simulink model "prj_2018a"  (R2018a)
settings: Solver=FixedStepAuto  StartTime=0.0  StopTime=T  FixedStep=0.01  RelTol=1e-3
values from neighbouring files (symbols this model uses):
  C0 = 0.008    [data.m]
  C1 = 1.6e-6    (= 1.6e-06)    [data.m]
  Cbat = 800    [data.m]
  Cx = 1.2    [data.m]
  D = 3    [data.m]
  g = 9.81    [data.m]
  m = 3    [data.m]
  rho = 1.225    [data.m]
  S = 0.0739    [data.m]
  T = 600    [data.m]
  VBAT = 12    [data.m]
libraries: simulink x3, powerlib_meascontrol x1
settings Model: Creator=xoxox  LastModifiedBy=eduhamel01
settings DataIOCC: ReturnWorkspaceOutputs=on
settings SFSimCC: SimUseLocalCustomCode=on
settings RTWCC: RTWUseLocalCustomCode=on

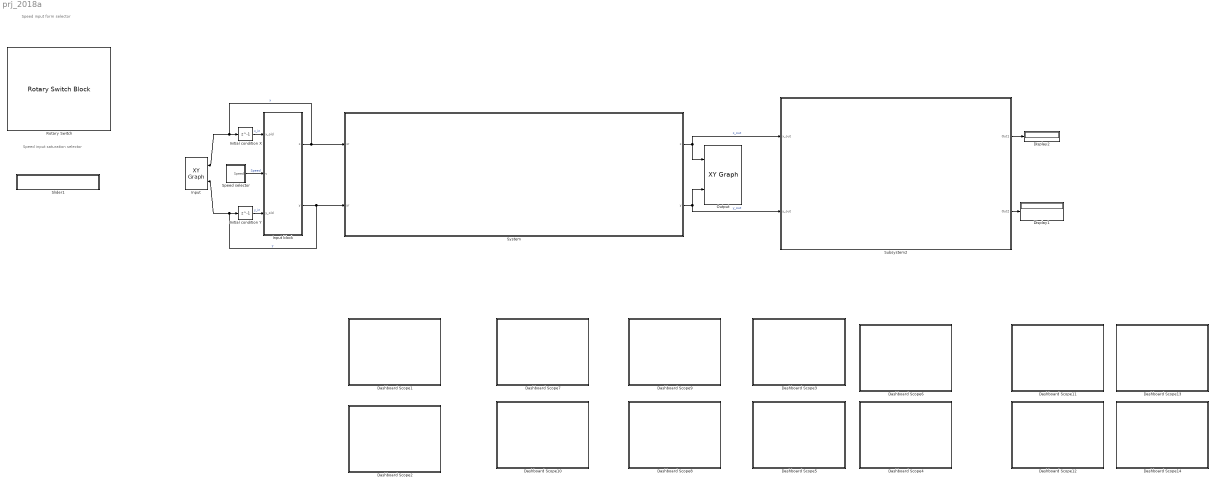
== system prj_2018a ==
  note: Speed input saturation
      | selector
  note: Speed input form selector
  Dashboard Scope1 : Subsystem  DialogController=hmiCreateDDGDialog  IsWebBlock=on  mask(MWDashboardBlock){webBlockId=119e8fbf-0f84-4c64-a065-49c5137ac74d, webBlockType=sdiscope, ShowInLibBrowser=on, ShowInitialText=on, HMISrcModelName=prj_2018a}
      mask prompts: webBlockId "WebBlock Id"; webBlockType "WebBlock Type"; HMISrcModelName "Source Model"
      mask help: Traces signals on the dashboard scope during simulation.
      mask Help: helpview([docroot '/mapfiles/simulink.map'], 'hmi_scope')
      mask Display:
      | if strcmp(get_param(bdroot(gcb),'BlockDiagramType'),'library')
      |  image([(matlabroot) '/toolbox/simulink/hmi/icons/SDIScope.png'])
      | end
  Dashboard Scope10 : Subsystem  DialogController=hmiCreateDDGDialog  IsWebBlock=on  mask(MWDashboardBlock){webBlockId=fa008d0d-197e-41b1-bb55-4dce241af62d, webBlockType=sdiscope, ShowInLibBrowser=on, ShowInitialText=on, HMISrcModelName=prj_2018a}
      mask prompts: webBlockId "WebBlock Id"; webBlockType "WebBlock Type"; HMISrcModelName "Source Model"
      mask help: Traces signals on the dashboard scope during simulation.
      mask Help: helpview([docroot '/mapfiles/simulink.map'], 'hmi_scope')
      mask Display:
      | if strcmp(get_param(bdroot(gcb),'BlockDiagramType'),'library')
      |  image([(matlabroot) '/toolbox/simulink/hmi/icons/SDIScope.png'])
      | end
  Dashboard Scope11 : Subsystem  DialogController=hmiCreateDDGDialog  IsWebBlock=on  mask(MWDashboardBlock){webBlockId=fa4fd851-4fca-4c18-b171-96f8acd06293, webBlockType=sdiscope, ShowInLibBrowser=on, ShowInitialText=on, HMISrcModelName=prj_2018a}
      mask prompts: webBlockId "WebBlock Id"; webBlockType "WebBlock Type"; HMISrcModelName "Source Model"
      mask help: Traces signals on the dashboard scope during simulation.
      mask Help: helpview([docroot '/mapfiles/simulink.map'], 'hmi_scope')
      mask Display:
      | if strcmp(get_param(bdroot(gcb),'BlockDiagramType'),'library')
      |  image([(matlabroot) '/toolbox/simulink/hmi/icons/SDIScope.png'])
      | end
  Dashboard Scope12 : Subsystem  DialogController=hmiCreateDDGDialog  IsWebBlock=on  mask(MWDashboardBlock){webBlockId=7913e7ce-348c-44da-9251-239d1fa42c28, webBlockType=sdiscope, ShowInLibBrowser=on, ShowInitialText=on, HMISrcModelName=prj_2018a}
      mask prompts: webBlockId "WebBlock Id"; webBlockType "WebBlock Type"; HMISrcModelName "Source Model"
      mask help: Traces signals on the dashboard scope during simulation.
      mask Help: helpview([docroot '/mapfiles/simulink.map'], 'hmi_scope')
      mask Display:
      | if strcmp(get_param(bdroot(gcb),'BlockDiagramType'),'library')
      |  image([(matlabroot) '/toolbox/simulink/hmi/icons/SDIScope.png'])
      | end
  Dashboard Scope13 : Subsystem  DialogController=hmiCreateDDGDialog  IsWebBlock=on  mask(MWDashboardBlock){webBlockId=8edd69cc-18a3-423d-a06d-795dad7adbdd, webBlockType=sdiscope, ShowInLibBrowser=on, ShowInitialText=on, HMISrcModelName=prj_2018a}
      mask prompts: webBlockId "WebBlock Id"; webBlockType "WebBlock Type"; HMISrcModelName "Source Model"
      mask help: Traces signals on the dashboard scope during simulation.
      mask Help: helpview([docroot '/mapfiles/simulink.map'], 'hmi_scope')
      mask Display:
      | if strcmp(get_param(bdroot(gcb),'BlockDiagramType'),'library')
      |  image([(matlabroot) '/toolbox/simulink/hmi/icons/SDIScope.png'])
      | end
  Dashboard Scope14 : Subsystem  DialogController=hmiCreateDDGDialog  IsWebBlock=on  mask(MWDashboardBlock){webBlockId=3235017e-418f-422e-8807-0662af4a4bf4, webBlockType=sdiscope, ShowInLibBrowser=on, ShowInitialText=on, HMISrcModelName=prj_2018a}
      mask prompts: webBlockId "WebBlock Id"; webBlockType "WebBlock Type"; HMISrcModelName "Source Model"
      mask help: Traces signals on the dashboard scope during simulation.
      mask Help: helpview([docroot '/mapfiles/simulink.map'], 'hmi_scope')
      mask Display:
      | if strcmp(get_param(bdroot(gcb),'BlockDiagramType'),'library')
      |  image([(matlabroot) '/toolbox/simulink/hmi/icons/SDIScope.png'])
      | end
  Dashboard Scope2 : Subsystem  DialogController=hmiCreateDDGDialog  IsWebBlock=on  mask(MWDashboardBlock){webBlockId=834b94e8-2ac5-4a88-9e83-ba3259317c2a, webBlockType=sdiscope, ShowInLibBrowser=on, ShowInitialText=on, HMISrcModelName=prj_2018a}
      mask prompts: webBlockId "WebBlock Id"; webBlockType "WebBlock Type"; HMISrcModelName "Source Model"
      mask help: Traces signals on the dashboard scope during simulation.
      mask Help: helpview([docroot '/mapfiles/simulink.map'], 'hmi_scope')
      mask Display:
      | if strcmp(get_param(bdroot(gcb),'BlockDiagramType'),'library')
      |  image([(matlabroot) '/toolbox/simulink/hmi/icons/SDIScope.png'])
      | end
  Dashboard Scope3 : Subsystem  DialogController=hmiCreateDDGDialog  IsWebBlock=on  mask(MWDashboardBlock){webBlockId=06c2f07c-ed11-4a51-95f8-aa5a8867ac83, webBlockType=sdiscope, ShowInLibBrowser=on, ShowInitialText=on, HMISrcModelName=prj_2018a}
      mask prompts: webBlockId "WebBlock Id"; webBlockType "WebBlock Type"; HMISrcModelName "Source Model"
      mask help: Traces signals on the dashboard scope during simulation.
      mask Help: helpview([docroot '/mapfiles/simulink.map'], 'hmi_scope')
      mask Display:
      | if strcmp(get_param(bdroot(gcb),'BlockDiagramType'),'library')
      |  image([(matlabroot) '/toolbox/simulink/hmi/icons/SDIScope.png'])
      | end
  Dashboard Scope4 : Subsystem  DialogController=hmiCreateDDGDialog  IsWebBlock=on  mask(MWDashboardBlock){webBlockId=6b045230-5b5a-4611-980b-31087ea3d308, webBlockType=sdiscope, ShowInLibBrowser=on, ShowInitialText=on, HMISrcModelName=prj_2018a}
      mask prompts: webBlockId "WebBlock Id"; webBlockType "WebBlock Type"; HMISrcModelName "Source Model"
      mask help: Traces signals on the dashboard scope during simulation.
      mask Help: helpview([docroot '/mapfiles/simulink.map'], 'hmi_scope')
      mask Display:
      | if strcmp(get_param(bdroot(gcb),'BlockDiagramType'),'library')
      |  image([(matlabroot) '/toolbox/simulink/hmi/icons/SDIScope.png'])
      | end
  Dashboard Scope5 : Subsystem  DialogController=hmiCreateDDGDialog  IsWebBlock=on  mask(MWDashboardBlock){webBlockId=d05e08e3-8fad-4b3c-942c-8af112444a54, webBlockType=sdiscope, ShowInLibBrowser=on, ShowInitialText=on, HMISrcModelName=prj_2018a}
      mask prompts: webBlockId "WebBlock Id"; webBlockType "WebBlock Type"; HMISrcModelName "Source Model"
      mask help: Traces signals on the dashboard scope during simulation.
      mask Help: helpview([docroot '/mapfiles/simulink.map'], 'hmi_scope')
      mask Display:
      | if strcmp(get_param(bdroot(gcb),'BlockDiagramType'),'library')
      |  image([(matlabroot) '/toolbox/simulink/hmi/icons/SDIScope.png'])
      | end
  Dashboard Scope6 : Subsystem  DialogController=hmiCreateDDGDialog  IsWebBlock=on  mask(MWDashboardBlock){webBlockId=a3c59839-8da6-40a2-abfa-24167c38daa9, webBlockType=sdiscope, ShowInLibBrowser=on, ShowInitialText=on, HMISrcModelName=prj_2018a}
      mask prompts: webBlockId "WebBlock Id"; webBlockType "WebBlock Type"; HMISrcModelName "Source Model"
      mask help: Traces signals on the dashboard scope during simulation.
      mask Help: helpview([docroot '/mapfiles/simulink.map'], 'hmi_scope')
      mask Display:
      | if strcmp(get_param(bdroot(gcb),'BlockDiagramType'),'library')
      |  image([(matlabroot) '/toolbox/simulink/hmi/icons/SDIScope.png'])
      | end
  Dashboard Scope7 : Subsystem  DialogController=hmiCreateDDGDialog  IsWebBlock=on  mask(MWDashboardBlock){webBlockId=a1a62eab-3a48-418c-ad90-13885701b78d, webBlockType=sdiscope, ShowInLibBrowser=on, ShowInitialText=on, HMISrcModelName=prj_2018a}
      mask prompts: webBlockId "WebBlock Id"; webBlockType "WebBlock Type"; HMISrcModelName "Source Model"
      mask help: Traces signals on the dashboard scope during simulation.
      mask Help: helpview([docroot '/mapfiles/simulink.map'], 'hmi_scope')
      mask Display:
      | if strcmp(get_param(bdroot(gcb),'BlockDiagramType'),'library')
      |  image([(matlabroot) '/toolbox/simulink/hmi/icons/SDIScope.png'])
      | end
  Dashboard Scope8 : Subsystem  DialogController=hmiCreateDDGDialog  IsWebBlock=on  mask(MWDashboardBlock){webBlockId=c0fb3f3b-45df-43b4-8987-c7cbfe6d8ce9, webBlockType=sdiscope, ShowInLibBrowser=on, ShowInitialText=on, HMISrcModelName=prj_2018a}
      mask prompts: webBlockId "WebBlock Id"; webBlockType "WebBlock Type"; HMISrcModelName "Source Model"
      mask help: Traces signals on the dashboard scope during simulation.
      mask Help: helpview([docroot '/mapfiles/simulink.map'], 'hmi_scope')
      mask Display:
      | if strcmp(get_param(bdroot(gcb),'BlockDiagramType'),'library')
      |  image([(matlabroot) '/toolbox/simulink/hmi/icons/SDIScope.png'])
      | end
  Dashboard Scope9 : Subsystem  DialogController=hmiCreateDDGDialog  IsWebBlock=on  mask(MWDashboardBlock){webBlockId=857b3752-856c-4ac0-8c31-3300ce0e1cd1, webBlockType=sdiscope, ShowInLibBrowser=on, ShowInitialText=on, HMISrcModelName=prj_2018a}
      mask prompts: webBlockId "WebBlock Id"; webBlockType "WebBlock Type"; HMISrcModelName "Source Model"
      mask help: Traces signals on the dashboard scope during simulation.
      mask Help: helpview([docroot '/mapfiles/simulink.map'], 'hmi_scope')
      mask Display:
      | if strcmp(get_param(bdroot(gcb),'BlockDiagramType'),'library')
      |  image([(matlabroot) '/toolbox/simulink/hmi/icons/SDIScope.png'])
      | end
  Display1 : Display
  Display2 : Display
  Initial condition X : Delay  DelayLength=1
  Initial condition Y : Delay  DelayLength=1
  Input : simulink/Sinks/XY Graph  xmin=-1  xmax=5.5  ymin=-5  ymax=20  st=-1
  Input block : MATLAB Function  TreatAsAtomicUnit=on
  Output : simulink/Sinks/XY Graph  xmin=-1  xmax=5.5  ymin=-5  ymax=20  st=-1
  Rotary Switch : RotarySwitchBlock  WebBlockId=65
      settings: Values={{'Constant', 'Sine', 'Pulse', 'Ramp', 'Triangle'}, [1 2 3 4 5]}
  Slider1 : Subsystem  DialogController=hmiCreateDDGDialog  IsWebBlock=on  mask(MWDashboardBlock){webBlockId=c1551613-8028-4e7c-bb00-03568ac3d875, webBlockType=slider, ShowInLibBrowser=on, ShowInitialText=on, HMISrcModelName=prj_2018a}
      mask prompts: webBlockId "WebBlock Id"; webBlockType "WebBlock Type"; HMISrcModelName "Source Model"
      mask help: Set value to tune parameters or variables.
      mask Help: helpview([docroot '/mapfiles/simulink.map'], 'hmi_slider')
      mask Display:
      | if strcmp(get_param(bdroot(gcb),'BlockDiagramType'),'library')
      |  image([(matlabroot) '/toolbox/simulink/hmi/icons/Slider.png'])
      | end
  Speed selector : Subsystem
  Subsystem2 : Subsystem
  System : Subsystem
  wires:
  System/1(x) -> Subsystem2/1(x_out), Output/1  "x_out"
  System/2(y) -> Subsystem2/2(y_out), Output/2  "y_out"
  Input block/2(y) -> Input/2, Initial condition Y/1, System/2(yr)  "y"
  Initial condition Y/1 -> Input block/3(y_old)  "y_in"
  Initial condition X/1 -> Input block/1(x_old)  "x_in"
  Input block/1(x) -> Initial condition X/1, Input/1, System/1(xr)  "x"
  Speed selector/1(Speed) -> Input block/2(v)  "Speed"
  Subsystem2/1(Out1) -> Display2/1
  Subsystem2/2(Out2) -> Display1/1

== system prj_2018a/Dashboard Scope1 ==

== system prj_2018a/Dashboard Scope10 ==

== system prj_2018a/Dashboard Scope11 ==

== system prj_2018a/Dashboard Scope12 ==

== system prj_2018a/Dashboard Scope13 ==

== system prj_2018a/Dashboard Scope14 ==

== system prj_2018a/Dashboard Scope2 ==

== system prj_2018a/Dashboard Scope3 ==

== system prj_2018a/Dashboard Scope4 ==

== system prj_2018a/Dashboard Scope5 ==

== system prj_2018a/Dashboard Scope6 ==

== system prj_2018a/Dashboard Scope7 ==

== system prj_2018a/Dashboard Scope8 ==

== system prj_2018a/Dashboard Scope9 ==

== system prj_2018a/Slider1 ==

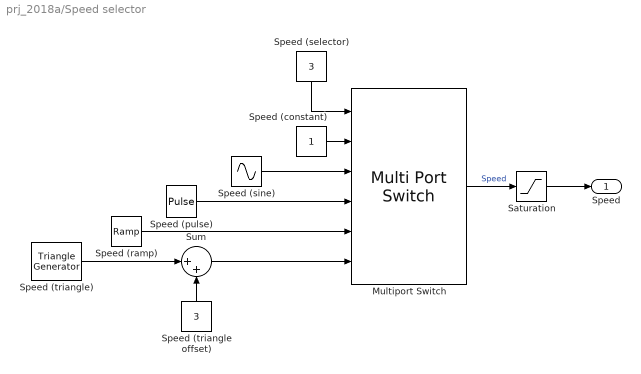
== system prj_2018a/Speed selector ==
  Multiport Switch : MultiPortSwitch  Inputs=5
  Saturation : Saturate  UpperLimit=4.664899955035971
  Speed (constant) : Constant
  Speed (pulse) : DiscretePulseGenerator  PulseType=Time based  Amplitude=0.1  Period=10  PulseWidth=50
  Speed (ramp) : simulink/Sources/Ramp  slope=1  start=0  InitialOutput=0
  Speed (selector) : Constant  Value=3
  Speed (sine) : Sin  Bias=1  SampleTime=0
  Speed (triangle offset) : Constant  Value=3
  Speed (triangle) : powerlib_meascontrol/Pulse & Signal Generators/Triangle Generator  Freq=1/30  Phase=90  Ts=0
  Sum : Sum  Inputs=|++
  Speed : Outport  VectorParamsAs1DForOutWhenUnconnected=on
  wires:
  Speed (triangle offset)/1 -> Sum/2
  Sum/1 -> Multiport Switch/6
  Speed (pulse)/1 -> Multiport Switch/4
  Speed (triangle)/1 -> Sum/1
  Speed (sine)/1 -> Multiport Switch/3
  Speed (constant)/1 -> Multiport Switch/2
  Speed (selector)/1 -> Multiport Switch/1
  Speed (ramp)/1 -> Multiport Switch/5
  Multiport Switch/1 -> Saturation/1  "Speed"
  Saturation/1 -> Speed/1

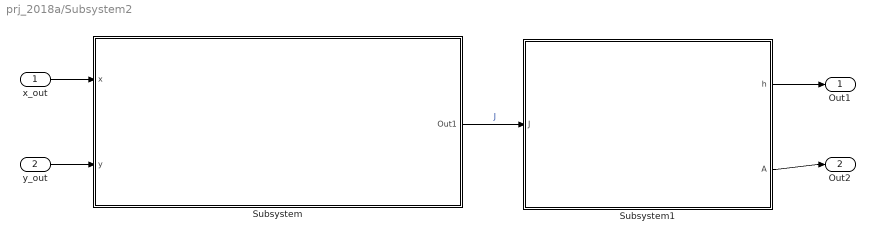
== system prj_2018a/Subsystem2 ==
  x_out : Inport
  y_out : Inport  Port=2
  Subsystem : Subsystem
  Subsystem1 : Subsystem
  Out1 : Outport
  Out2 : Outport  Port=2
  wires:
  Subsystem/1(Out1) -> Subsystem1/1(J)  "J"
  Subsystem1/2(A) -> Out2/1
  y_out/1 -> Subsystem/2(y)
  Subsystem1/1(h) -> Out1/1
  x_out/1 -> Subsystem/1(x)

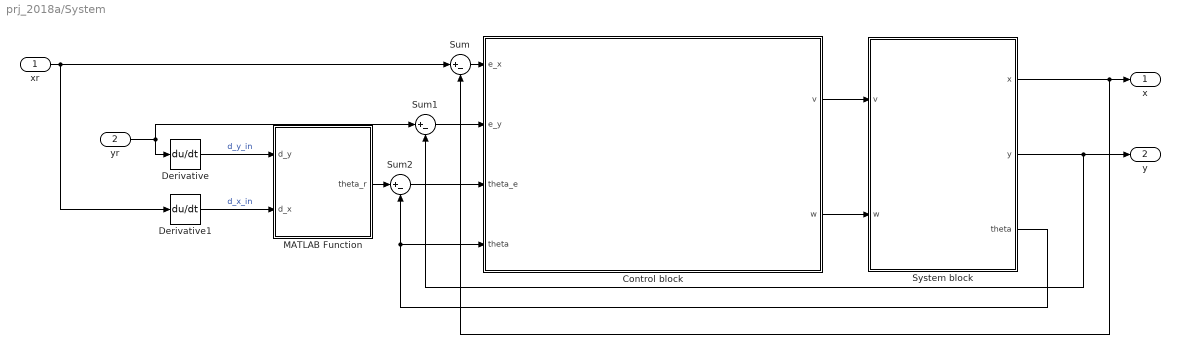
== system prj_2018a/System ==
  xr : Inport
  yr : Inport  Port=2
  Control block : Subsystem
  Derivative : Derivative
  Derivative1 : Derivative
  MATLAB Function : MATLAB Function  TreatAsAtomicUnit=on
  Sum : Sum  Inputs=|+-
  Sum1 : Sum  Inputs=|+-
  Sum2 : Sum  Inputs=|+-
  System block : Subsystem
  x : Outport
  y : Outport  Port=2
  wires:
  Sum1/1 -> Control block/2(e_y)
  Control block/2(w) -> System block/2(w)
  Derivative/1 -> MATLAB Function/1(d_y)  "d_y_in"
  MATLAB Function/1(theta_r) -> Sum2/1
  System block/2(y) -> y/1, Sum1/2
  System block/3(theta) -> Control block/4(theta), Sum2/2
  System block/1(x) -> x/1, Sum/2
  Derivative1/1 -> MATLAB Function/2(d_x)  "d_x_in"
  Sum/1 -> Control block/1(e_x)
  Control block/1(v) -> System block/1(v)
  Sum2/1 -> Control block/3(theta_e)
  yr/1 -> Derivative/1, Sum1/1
  xr/1 -> Sum/1, Derivative1/1

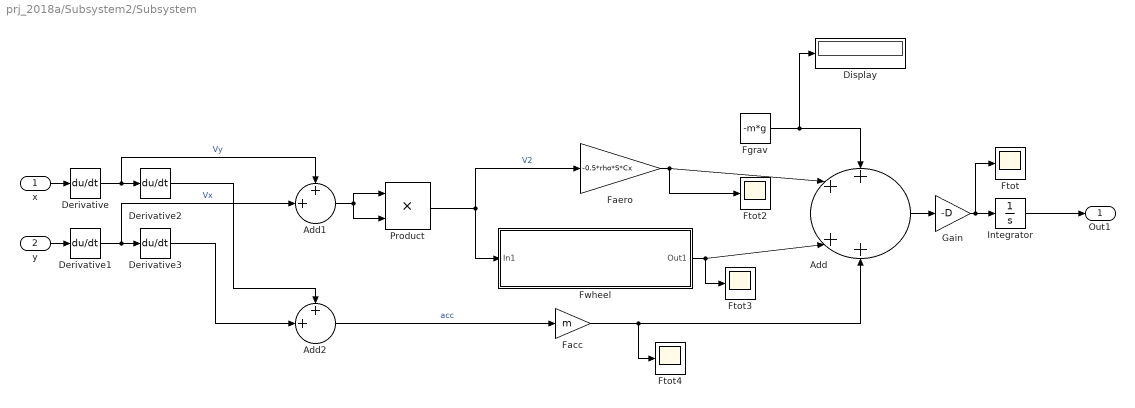
== system prj_2018a/Subsystem2/Subsystem ==
  x : Inport
  y : Inport  Port=2
  Add : Sum  Inputs=++|++
  Add1 : Sum  Inputs=++|
  Add2 : Sum  Inputs=++|
  Derivative{,1..3} (4 alike) : Derivative
  Display : Display
  Facc : Gain  Gain=m
  Faero : Gain  Gain=-0.5*rho*S*Cx
  Fgrav : Constant  Value=-m*g
  Ftot{,2..4} (4 alike) : Scope
  Fwheel : Subsystem
  Gain : Gain  Gain=-D
  Integrator : Integrator
  Product : Product
  Out1 : Outport  VectorParamsAs1DForOutWhenUnconnected=on
  wires:
  Derivative/1 -> Add1/1, Derivative2/1  "Vy"
  Faero/1 -> Ftot2/1, Add/2
  Add2/1 -> Facc/1  "acc"
  Product/1 -> Faero/1, Fwheel/1(In1)  "V2"
  Derivative1/1 -> Add1/2, Derivative3/1  "Vx"
  Derivative3/1 -> Add2/2
  Gain/1 -> Integrator/1, Ftot/1
  Derivative2/1 -> Add2/1
  Fgrav/1 -> Display/1, Add/1
  Add/1 -> Gain/1
  Facc/1 -> Ftot4/1, Add/4
  Add1/1 -> Product/1, Product/2
  y/1 -> Derivative1/1
  x/1 -> Derivative/1
  Integrator/1 -> Out1/1
  Fwheel/1(Out1) -> Add/3, Ftot3/1

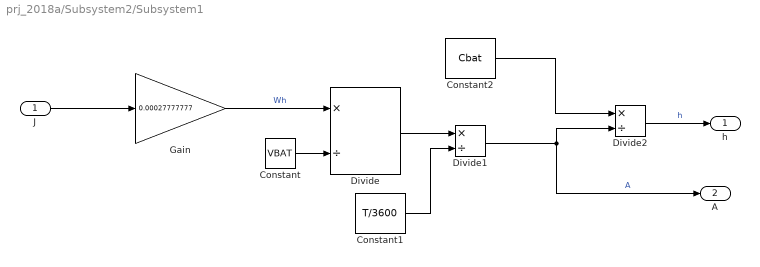
== system prj_2018a/Subsystem2/Subsystem1 ==
  J : Inport
  Constant : Constant  Value=VBAT
  Constant1 : Constant  Value=T/3600
  Constant2 : Constant  Value=Cbat
  Divide : Product  Inputs=*/
  Divide1 : Product  Inputs=*/
  Divide2 : Product  Inputs=*/
  Gain : Gain  Gain=0.00027777777
  h : Outport
  A : Outport  Port=2
  wires:
  Divide2/1 -> h/1  "h"
  Constant2/1 -> Divide2/1
  Constant/1 -> Divide/2
  Divide1/1 -> A/1, Divide2/2  "A"
  Gain/1 -> Divide/1  "Wh"
  Constant1/1 -> Divide1/2
  Divide/1 -> Divide1/1
  J/1 -> Gain/1

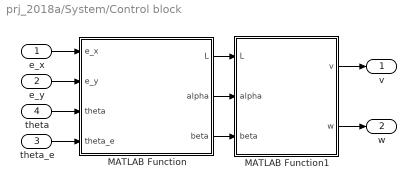
== system prj_2018a/System/Control block ==
  e_x : Inport
  e_y : Inport  Port=2
  theta_e : Inport  Port=3
  theta : Inport  Port=4
  MATLAB Function : MATLAB Function  TreatAsAtomicUnit=on
  MATLAB Function1 : MATLAB Function  TreatAsAtomicUnit=on
  v : Outport
  w : Outport  Port=2
  wires:
  MATLAB Function1/1(v) -> v/1
  MATLAB Function1/2(w) -> w/1
  e_x/1 -> MATLAB Function/1(e_x)
  e_y/1 -> MATLAB Function/2(e_y)
  theta_e/1 -> MATLAB Function/4(theta_e)
  MATLAB Function/1(L) -> MATLAB Function1/1(L)
  MATLAB Function/2(alpha) -> MATLAB Function1/2(alpha)
  MATLAB Function/3(beta) -> MATLAB Function1/3(beta)
  theta/1 -> MATLAB Function/3(theta)

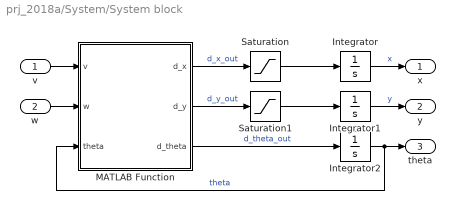
== system prj_2018a/System/System block ==
  v : Inport
  w : Inport  Port=2
  Integrator : Integrator
  Integrator1 : Integrator
  Integrator2 : Integrator
  MATLAB Function : MATLAB Function  TreatAsAtomicUnit=on
  Saturation : Saturate  UpperLimit=0.33  LowerLimit=-0.33
  Saturation1 : Saturate  UpperLimit=0.33  LowerLimit=-0.33
  x : Outport
  y : Outport  Port=2
  theta : Outport  Port=3
  wires:
  Integrator2/1 -> theta/1, MATLAB Function/3(theta)  "theta"
  MATLAB Function/3(d_theta) -> Integrator2/1  "d_theta_out"
  v/1 -> MATLAB Function/1(v)
  Integrator/1 -> x/1  "x"
  w/1 -> MATLAB Function/2(w)
  Integrator1/1 -> y/1  "y"
  MATLAB Function/1(d_x) -> Saturation/1  "d_x_out"
  Saturation/1 -> Integrator/1
  MATLAB Function/2(d_y) -> Saturation1/1  "d_y_out"
  Saturation1/1 -> Integrator1/1

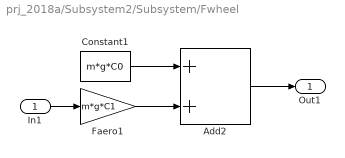
== system prj_2018a/Subsystem2/Subsystem/Fwheel ==
  In1 : Inport
  Add2 : Sum
  Constant1 : Constant  Value=m*g*C0
  Faero1 : Gain  Gain=m*g*C1
  Out1 : Outport  VectorParamsAs1DForOutWhenUnconnected=on
  wires:
  Faero1/1 -> Add2/2
  Add2/1 -> Out1/1
  Constant1/1 -> Add2/1
  In1/1 -> Faero1/1

== matlab function prj_2018a/System/Control block/MATLAB Function ==
  data: e_x input; L output; e_y input; theta input; theta_e input; alpha output; beta output
function [L , alpha, beta] = to_parameters(e_x , e_y , theta , theta_e)
    L = sqrt(e_x * e_x + e_y * e_y);
    alpha = mod(atan2(e_y , e_x) , 2*pi) - theta;
    beta = theta_e - alpha;
end

== matlab function prj_2018a/System/System block/MATLAB Function ==
  data: v input; d_x output; w input; theta input; d_y output; d_theta output
function [d_x,  d_y,  d_theta] = system(v , w , theta)

    d_x = v*cos(theta);
    d_y = v*sin(theta);
    d_theta = w;

end

== matlab function prj_2018a/System/Control block/MATLAB Function1 ==
  data: L input; v output; w output; alpha input; beta input
function [v , w] = to_v_w(L, alpha , beta)

%old
% k_L = -3;
% k_alpha = -210;
% k_beta = 4.5;


k_L = -5.5;
k_alpha = -220;
k_beta = 2;

v = -k_L * L;
w = -k_alpha * alpha - k_beta * beta;

end

== matlab function prj_2018a/System/MATLAB Function ==
  data: d_y input; d_x input; theta_r output
function theta_r = arctan2(d_y , d_x)
    theta_r = mod(atan2(d_y , d_x) , 2*pi);
end

== matlab function prj_2018a/Input block ==
  data: x output; x_old input; v input; y_old input; y output
function [x, y] = input(x_old , v , y_old)

    h = 10; %Straight line distance
    d = 5; %"Circle" diameter
    
    Ts = 0.01; %MUST also Simulink sample time

    is_on_part_1_flag = ((x_old == 0 && y_old < h));
    is_on_part_2_flag = ((x_old < d && y_old >= h));
    is_on_part_3_flag = ((x_old >= d && y_old >=0));
    is_on_part_4_flag = (~is_on_part_1_flag &&...
                         ~is_on_part_2_flag &&...
                         ~is_on_part_3_flag);
  
                     
         
    x = is_on_part_1_flag * (0)+...
        is_on_part_2_flag * (x_old + Ts*v)+... 
        is_on_part_3_flag * (d)+...
        is_on_part_4_flag * ((x_old - Ts*v > 0)*(x_old - Ts*v)); %Ternary operator workaround

    y = is_on_part_1_flag * (y_old + Ts*v)+...
        is_on_part_2_flag * (h + (d/2)*sin(pi*x/d))+... 
        is_on_part_3_flag * (y_old - Ts*v)+...
        is_on_part_4_flag * (- (d/2)*sin(pi*x/d));    

         
%     x = is_on_part_1_flag * (0)+...
%         is_on_part_2_flag * (timestamp*v)+... 
%         is_on_part_3_flag * (d)+...
%         is_on_part_4_flag * ((d - timestamp*v >0)*(d - timestamp*v));
%    
%     y = is_on_part_1_flag * (timestamp*v)+...
%         is_on_part_2_flag * (h + (d/2) * sin(pi*timestamp*v/d))+... 
%         is_on_part_3_flag * (h-timestamp*v)+...
%         is_on_part_4_flag * (-(d/2) * sin(pi*timestamp*v/d));
 

            
            


end
